simulink model "MPC_multiFeed"  (R2022a)
settings: Solver=VariableStepAuto  StartTime=0.0  StopTime=240  RelTol=1e-3
values from neighbouring files (symbols this model uses):
  Tf = 240    [plotConstFeed.m]    (also in plotMultiFeed.m; plotSimulinkLog.m; plotSingleFeed.m)
undefined symbols (not defined in the file or in its folder): N, Ts, x0
libraries: mpclib x1
settings Model: Creator=tomok  LastModifiedBy=tomok

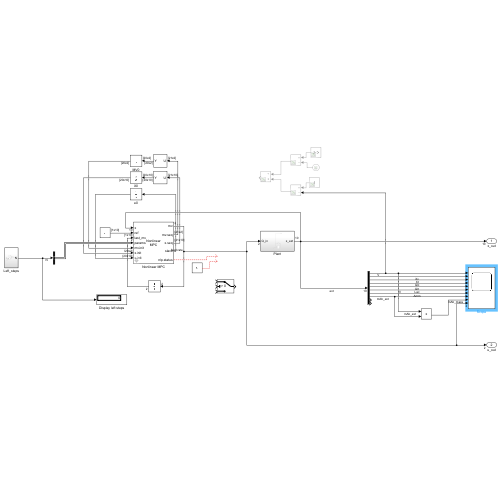
[thumbnail: Simulink's stored preview of the top-level diagram]
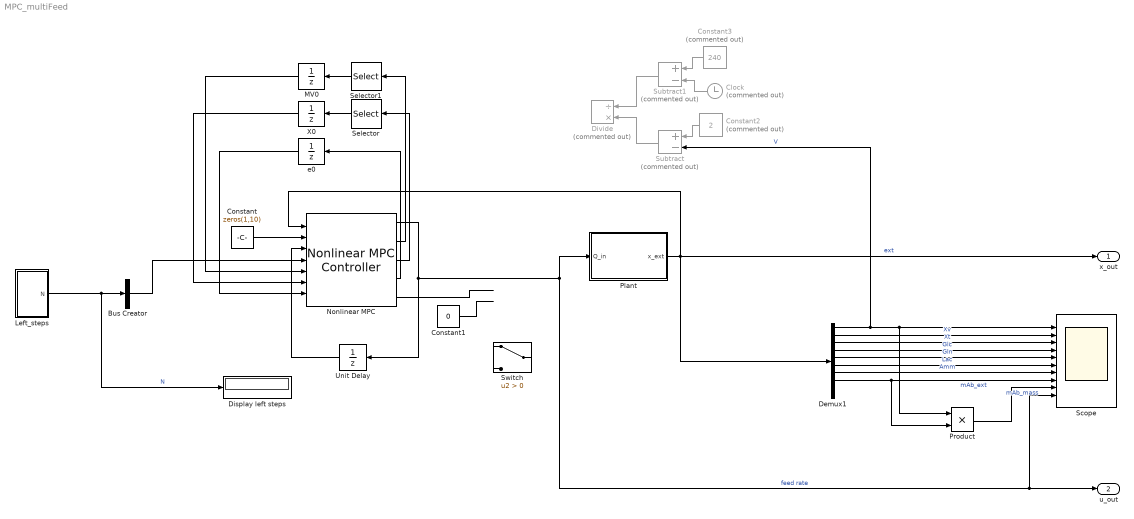
== system MPC_multiFeed ==
  Bus Creator : BusCreator  Inputs=1  OutDataTypeStr=Bus: myBusObject  NonVirtualBus=on
      settings: InheritFromInputs=off
  Clock : Clock  Commented=on
  Constant : Constant  Value=zeros(1,10)  VectorParams1D=off
  Constant1 : Constant  Value=0
  Constant2 : Constant  Commented=on  Value=2
  Constant3 : Constant  Commented=on  Value=240
  Demux1 : Demux  Outputs=10
  Display left steps : Display
  Divide : Product  Commented=on  Inputs=/*
  Left_steps : Subsystem
  MV0 : UnitDelay  InitialCondition=Info_error.MVopt(2:end,:)  SampleTime=-1  HasFrameUpgradeWarning=on
  Nonlinear MPC : mpclib/Nonlinear MPC Controller  nlmpcobj=nlmpcClosedLoop  UseObjectTs=on  UseMEX=off  md_enabled=off  mvtarget_enabled=off  param_enabled=on  cost_enabled=off  mvseq_enabled=on  stateseq_enabled=on  ovseq_enabled=off  slack_enabled=on  status_enabled=on  ov_min=off  ov_max=off  mv_min=off  mv_max=off  mvrate_min=off  mvrate_max=off  state_min=off  state_max=off  ov_weight=off  mv_weight=off  mvrate_weight=off  ecr_weight=off  nlp_initialize=on
  Plant : Subsystem
  Product : Product
  Scope : Scope  NumInputPorts=10
  Selector : Selector  NumberOfDimensions=2  InputPortWidth=3  IndexOptions=Index vector (dialog),Select all  Indices=2:21,1  OutputSizes=1,1
  Selector1 : Selector  NumberOfDimensions=2  InputPortWidth=3  IndexOptions=Index vector (dialog),Select all  Indices=2:21,1  OutputSizes=1,1
  Subtract : Sum  Commented=on  Inputs=+-
  Subtract1 : Sum  Commented=on  Inputs=+-
  Switch : Switch  Criteria=u2 > Threshold  SaturateOnIntegerOverflow=off  InputSameDT=off
  Unit Delay : UnitDelay  InitialCondition=1/Tf*[1;1]  SampleTime=-1  HasFrameUpgradeWarning=on
  X0 : UnitDelay  InitialCondition=Info_error.Xopt(2:end,:)  SampleTime=-1  HasFrameUpgradeWarning=on
  e0 : UnitDelay  SampleTime=-1  HasFrameUpgradeWarning=on
  x_out : Outport
  u_out : Outport  Port=2
  wires:
  Nonlinear MPC/1 -> u_out/1, Scope/10, Plant/1(Q_in), Unit Delay/1  "feed rate"
  Constant/1 -> Nonlinear MPC/2
  Unit Delay/1 -> Nonlinear MPC/3
  Bus Creator/1 -> Nonlinear MPC/4
  Left_steps/1(N) -> Bus Creator/1, Display left steps/1  "N"
  Product/1 -> Scope/9  "mAb_mass"
  Demux1/4 -> Scope/4  "Glc"
  Demux1/8 -> Product/2, Scope/8  "mAb_ext"
  Demux1/1 -> Subtract/2, Product/1, Scope/1  "V"
  Demux1/5 -> Scope/5  "Gln"
  Demux1/3 -> Scope/3  "Xt"
  Plant/1(x_ext) -> Demux1/1, x_out/1, Nonlinear MPC/1  "ext"
  Demux1/6 -> Scope/6  "Lac"
  Demux1/7 -> Scope/7  "Amm"
  Demux1/2 -> Scope/2  "Xv"
  Nonlinear MPC/2 -> Selector1/1
  MV0/1 -> Nonlinear MPC/5
  Nonlinear MPC/3 -> Selector/1
  X0/1 -> Nonlinear MPC/6
  Nonlinear MPC/4 -> e0/1
  Selector/1 -> X0/1
  Selector1/1 -> MV0/1
  Nonlinear MPC/5 -> ?
  Constant1/1 -> ?
  Constant2/1 -> Subtract/1
  Clock/1 -> Subtract1/2
  Constant3/1 -> Subtract1/1
  Subtract1/1 -> Divide/1
  Subtract/1 -> Divide/2
  e0/1 -> Nonlinear MPC/7

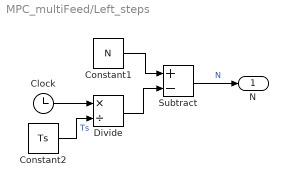
== system MPC_multiFeed/Left_steps ==
  Clock : Clock
  Constant1 : Constant  Value=N
  Constant2 : Constant  Value=Ts
  Divide : Product  Inputs=*/
  Subtract : Sum  Inputs=+-
  N : Outport
  wires:
  Constant2/1 -> Divide/2  "Ts"
  Divide/1 -> Subtract/2
  Clock/1 -> Divide/1
  Subtract/1 -> N/1  "N"
  Constant1/1 -> Subtract/1

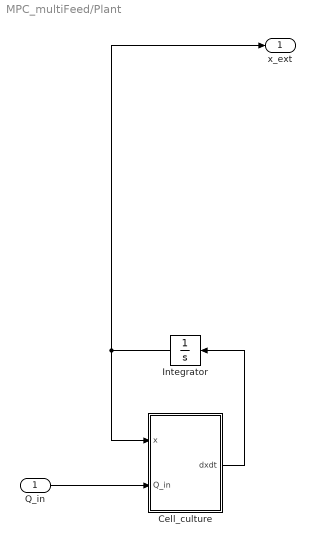
== system MPC_multiFeed/Plant ==
  Q_in : Inport
  Cell_culture : MATLAB Function  TreatAsAtomicUnit=on
  Integrator : Integrator  InitialCondition=x0  LimitOutput=on  LowerSaturationLimit=0
  x_ext : Outport
  wires:
  Cell_culture/1(dxdt) -> Integrator/1
  Q_in/1 -> Cell_culture/2(Q_in)
  Integrator/1 -> x_ext/1, Cell_culture/1(x)

== matlab function MPC_multiFeed/Plant/Cell_culture ==
  data: dxdt output; x input; Q_in input
function dxdt = fcn(x,Q_in)
dxdt = deTremblay1992MFStateFcn(x,Q_in);
end
